simulink model "experimental_setup_AIF"  (R2013b)
settings: Solver=ode45  StartTime=0.0  StopTime=6  FixedStep=0.001  MaxStep=1e-3  RelTol=1e-4
InitFcn:
  | init_experimental_setup
undefined symbols (not defined in the file): dimSquareMatrix
libraries: LibraryExperimental x10
settings Model: Creator=steffen  LastModifiedBy=smauch
settings SolverCC: AutoInsertRateTranBlk=on
settings DataIOCC: SignalLoggingSaveFormat=ModelDataLogs
settings OptimizationCC: ExpressionDepthLimit=2147483647
settings DebuggingCC: StateNameClashWarn=warning
settings HardwareCC: ProdHWDeviceType=Generic->Unspecified (assume 32-bit Generic)
settings GRTTargetCC: CombineOutputUpdateFcns=off  GRTInterface=on

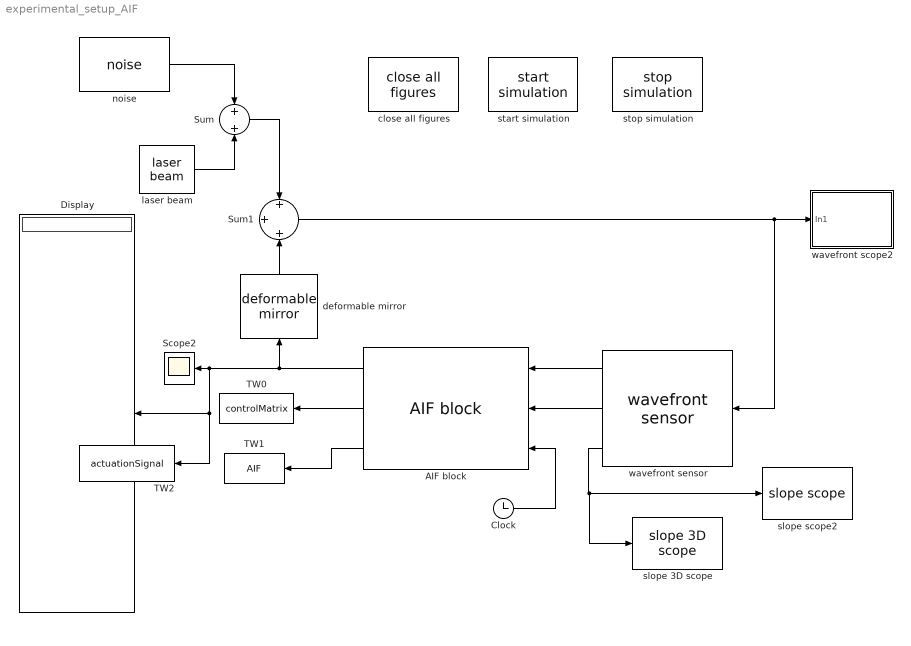
== system experimental_setup_AIF ==
  AIF block : LibraryExperimental/AIF block  nbAct=24
  Clock : Clock
      settings: Decimation=100
  Display : Display
  Scope2 : Scope
      settings: TimeRange=0.07317073170731714  YMin=-0.45  YMax=0.65  SaveName=ScopeData3
  Sum : Sum  Inputs=+|+
  Sum1 : Sum  Inputs=+|+|+
  TW0 : ToWorkspace  VariableName=controlMatrix  SampleTime=-1  SaveFormat=Timeseries
      settings: MaxDataPoints=10
  TW1 : ToWorkspace  VariableName=AIF  SampleTime=-1  SaveFormat=Timeseries
      settings: MaxDataPoints=10
  TW2 : ToWorkspace  VariableName=actuationSignal  SampleTime=-1  SaveFormat=Timeseries
  close all figures : LibraryExperimental/close all figures  SystemSampleTime=-1
  deformable mirror : LibraryExperimental/deformable mirror  dimActuator=dimActuator  dimMatrix=dimSquareMatrix  layoutActuator=layoutActuator  model=DMmodel
  laser beam : LibraryExperimental/laser beam  dimSquare=dimSquareMatrix
  noise : LibraryExperimental/noise  enable=on  dimSquare=dimSquareMatrix  Ts=1/2000  scaleNoise=25
  slope 3D scope : LibraryExperimental/slope 3D scope  sampleTime=0.025  dimMatrix=dimSlopeMatrix  enable=on  title='3D wavefront sensor'
  slope scope2 : LibraryExperimental/slope scope  sampleTime=0.1  dimMatrix=dimSlopeMatrix  enable=on  title='wavefront sensor'
  start simulation : LibraryExperimental/start simulation  SystemSampleTime=-1
  stop simulation : LibraryExperimental/stop simulation  SystemSampleTime=-1
  wavefront scope2 : Subsystem  mask{sampleTime=0.1, dimMatrix=dimSquareMatrix, enable=on, title='laser beam'}
      mask prompts: sampleTime "Sample Time"; dimMatrix "dimSquareMatrix"; enable "enable Scope"
      mask Display:
      | patch([0 0.5 1], [0 1 0],[1 0 0])
      | patch( [0.15 0.85 0.85 0.15], [0.6 0.6 0.4 0.4], [0.9 0.9 0.9] )
      | fprintf('Scope surf')
  wavefront sensor : LibraryExperimental/wavefront sensor  sampleTime=sampleTimeWavefrontSensor  dimMatrix_i=dimSquareMatrix  dimMatrix_o=dimSlopeMatrix  delay=delayWavefront  noiseSHWFS=1/128  scaleSHWFS=1/100  aperture=on
  wires:
  laser beam/1 -> Sum/2
  Sum/1 -> Sum1/1
  wavefront sensor/3 -> slope 3D scope/1, slope scope2/1
  deformable mirror/1 -> Sum1/3
  wavefront sensor/2 -> AIF block/2
  wavefront sensor/1 -> AIF block/1
  Clock/1 -> AIF block/3
  Sum1/1 -> wavefront scope2/1(In1), wavefront sensor/1
  AIF block/1 -> deformable mirror/1, Display/1, TW2/1, Scope2/1
  AIF block/2 -> TW0/1
  AIF block/3 -> TW1/1
  noise/1 -> Sum/1

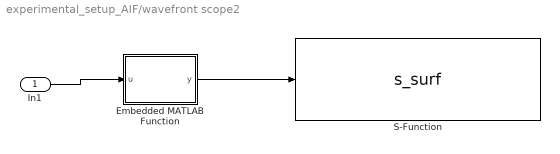
== system experimental_setup_AIF/wavefront scope2 ==
  In1 : Inport
  Embedded MATLAB Function : MATLAB Function  TreatAsAtomicUnit=on
  S-Function : S-Function  FunctionName=s_surf  Parameters=sampleTime,dimMatrix,enable,title  EnableBusSupport=off
  wires:
  Embedded MATLAB Function/1(y) -> S-Function/1
  In1/1 -> Embedded MATLAB Function/1(u)

== matlab function experimental_setup_AIF/wavefront scope2/Embedded MATLAB Function ==
  data: u input; y output
function y = fcn(u)
%#eml

y = u(:);
